simulink model "DT_LPV_sim"  (R2020b)
settings: Solver=VariableStepAuto  StartTime=0.0  StopTime=10.0  RelTol=1e-3
values from neighbouring files (symbols this model uses):
  a = -1    [simulink_generation.m]
  b = 1    [simulink_generation.m]
  K = 1:k_max    [DT_LPV_sim_script.m]    (also in simulink_generation.m = place(A,B, [-1+j,-1-j]))
libraries: cstblocks x2
settings Model: Creator=Jonas  LastModifiedBy=Jonas

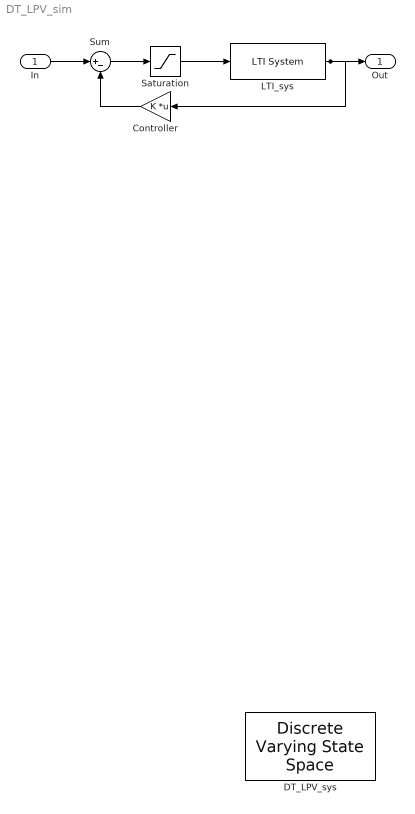
== system DT_LPV_sim ==
  In : Inport
  Controller : Gain  Gain=K  Multiplication=Matrix(K*u)
  DT_LPV_sys : cstblocks/Linear Parameter Varying/Discrete Varying State Space  x0=0  Ts=-1  OutputX=on  OutputDX=on
      settings: SourceProductBaseCode=CT
  LTI_sys : cstblocks/LTI System  sys=lti_sys  IC=x0
  Saturation : Saturate  UpperLimit=b  LowerLimit=a
  Sum : Sum  Inputs=|+-
  Out : Outport
  wires:
  Sum/1 -> Saturation/1
  Controller/1 -> Sum/2
  Saturation/1 -> LTI_sys/1
  In/1 -> Sum/1
  LTI_sys/1 -> Controller/1, Out/1
